simulink model "Simulink"  (R2019b)
settings: Solver=FixedStepAuto  StartTime=0.0  StopTime=5  FixedStep=0.001  RelTol=1e-3
values from neighbouring files (symbols this model uses):
  Awn0 = [0 1; -(wn0^2) -2*wn0*ounce]    [Autonomous_system_simulation.m]    (also in Autonomous_system_simulation_wsimulink.m)
  Awn1 = [0 1; -(wn1^2) -2*wn1*ounce]    [Autonomous_system_simulation.m]    (also in Autonomous_system_simulation_wsimulink.m)
  Awn2 = [0 1; -(wn2^2) -2*wn2*ounce]    [Autonomous_system_simulation.m]    (also in Autonomous_system_simulation_wsimulink.m)
  Awn3 = [0 1; -(wn3^2) -2*wn3*ounce]    [Autonomous_system_simulation.m]    (also in Autonomous_system_simulation_wsimulink.m)
  Cwn0 = [1 0; 0 1]    [Autonomous_system_simulation.m]    (also in Autonomous_system_simulation_wsimulink.m)
  Cwn2 = [1 0; 0 1]    [Autonomous_system_simulation.m]    (also in Autonomous_system_simulation_wsimulink.m)
  Cwn3 = [1 0; 0 1]    [Autonomous_system_simulation.m]    (also in Autonomous_system_simulation_wsimulink.m)
  Dwn0 = [0; 0]    [Autonomous_system_simulation.m]    (also in Autonomous_system_simulation_wsimulink.m)
  Gwn0 = [0; wn0^2]    [Autonomous_system_simulation.m]    (also in Autonomous_system_simulation_wsimulink.m)
  R = eye(2, 2)    [Autonomous_system_simulation.m]    (also in Autonomous_system_simulation_wsimulink.m)
undefined symbols (not defined in the file or in its folder): Continuous, Time
libraries: ctrlSharedLib x3
settings Model: Creator=HP  LastModifiedBy=Bekircan Keceoglu
settings DataIOCC: ReturnWorkspaceOutputs=off
settings DebuggingCC: ArithmeticOperatorsInVariantConditions=warning
settings SFSimCC: CustomCodeUndefinedFunction=UseInterfaceOnly

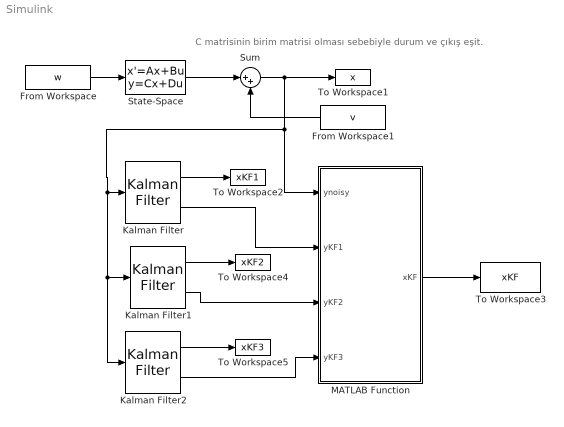
== system Simulink ==
  note: C matrisinin birim matrisi olması sebebiyle durum ve çıkış eşit.
  From Workspace : FromWorkspace  VariableName=w
  From Workspace1 : FromWorkspace  VariableName=v
  Kalman Filter : ctrlSharedLib/Kalman Filter  TimeDomain=Continuous-Time  UseCurrentEstimator=on  ModelSource=Individual A, B, C, D matrices  ModelSourceVariable=ss(0.95,1,1,0,1)  A=Awn1  B=[0;0.25]  C=Awn1  D=[0;0]  NumberOfStates=1  NumberOfInputs=1  NumberOfOutputs=1  InitialEstimateSource=Dialog  X0=0  P0=10  UseK=off  UseGH=on  NumberOfProcessNoiseInputs=1  G=Gwn1  TimeInvariantG=on  H=0  TimeInvariantH=on  Q=Q  TimeInvariantQ=on  R=R  TimeInvariantR=on  N=0  TimeInvariantN=on  AddInputPort=off  AddEnablePort=off  OutputEstimatedY=on  OutputP=off  Ts=-1
      settings: SourceProductBaseCode=CT
  Kalman Filter1 : ctrlSharedLib/Kalman Filter  TimeDomain=Continuous-Time  UseCurrentEstimator=on  ModelSource=Individual A, B, C, D matrices  ModelSourceVariable=ss(0.95,1,1,0,1)  A=Awn2  B=[0;100]  C=Cwn2  D=[0;0]  NumberOfStates=1  NumberOfInputs=1  NumberOfOutputs=1  InitialEstimateSource=Dialog  X0=0  P0=10  UseK=off  UseGH=on  NumberOfProcessNoiseInputs=1  G=Gwn2  TimeInvariantG=on  H=0  TimeInvariantH=on  Q=Q  TimeInvariantQ=on  R=R  TimeInvariantR=on  N=0  TimeInvariantN=on  AddInputPort=off  AddEnablePort=off  OutputEstimatedY=on  OutputP=off  Ts=-1
      settings: SourceProductBaseCode=CT
  Kalman Filter2 : ctrlSharedLib/Kalman Filter  TimeDomain=Continuous-Time  UseCurrentEstimator=on  ModelSource=Individual A, B, C, D matrices  ModelSourceVariable=ss(0.95,1,1,0,1)  A=Awn3  B=[0;625]  C=Cwn3  D=[0;0]  NumberOfStates=1  NumberOfInputs=1  NumberOfOutputs=1  InitialEstimateSource=Dialog  X0=0  P0=10  UseK=off  UseGH=on  NumberOfProcessNoiseInputs=1  G=Gwn3  TimeInvariantG=on  H=0  TimeInvariantH=on  Q=Q  TimeInvariantQ=on  R=R  TimeInvariantR=on  N=0  TimeInvariantN=on  AddInputPort=off  AddEnablePort=off  OutputEstimatedY=on  OutputP=off  Ts=-1
      settings: SourceProductBaseCode=CT
  MATLAB Function : MATLAB Function  TreatAsAtomicUnit=on
  State-Space : StateSpace  A=Awn0  B=Gwn0  C=Cwn0  D=Dwn0  InitialCondition=[1;10]
  Sum : Sum  Inputs=|++
  To Workspace1 : ToWorkspace  VariableName=x  SaveFormat=Timeseries  SampleTime=-1
  To Workspace2 : ToWorkspace  VariableName=xKF1  SaveFormat=Timeseries  SampleTime=-1
  To Workspace3 : ToWorkspace  VariableName=xKF  SaveFormat=Timeseries  SampleTime=-1
  To Workspace4 : ToWorkspace  VariableName=xKF2  SaveFormat=Timeseries  SampleTime=-1
  To Workspace5 : ToWorkspace  VariableName=xKF3  SaveFormat=Timeseries  SampleTime=-1
  wires:
  From Workspace/1 -> State-Space/1
  State-Space/1 -> Sum/1
  From Workspace1/1 -> Sum/2
  MATLAB Function/1(xKF) -> To Workspace3/1
  Sum/1 -> To Workspace1/1, MATLAB Function/1(ynoisy), Kalman Filter2/1, Kalman Filter1/1, Kalman Filter/1
  Kalman Filter/1 -> To Workspace2/1
  Kalman Filter1/1 -> To Workspace4/1
  Kalman Filter2/1 -> To Workspace5/1
  Kalman Filter/2 -> MATLAB Function/2(yKF1)
  Kalman Filter1/2 -> MATLAB Function/3(yKF2)
  Kalman Filter2/2 -> MATLAB Function/4(yKF3)

== matlab function Simulink/MATLAB Function ==
  data: ynoisy input; xKF output; yKF1 input; yKF2 input; yKF3 input
function xKF= decision_maker(ynoisy, yKF1, yKF2, yKF3)

% init xKF
xKF = [0; 0];

% error = (filterO(1) - systemO(1))^2 + (filterO(2) - systemO(2))^2 
eKF1 = (yKF1(1) - ynoisy(1))^2 + (yKF1(2) - ynoisy(2))^2 ;
eKF2 = (yKF2(1) - ynoisy(1))^2 + (yKF2(2) - ynoisy(2))^2 ;
eKF3 = (yKF3(1) - ynoisy(1))^2 + (yKF3(2) - ynoisy(2))^2 ;

% find min error
if ( eKF1 < eKF2 && eKF1 < eKF3 )
    xKF(1) = yKF1(1);
    xKF(2) = yKF1(2);
elseif ( eKF2 < eKF1 && eKF2 < eKF3 )
    xKF(1) = yKF2(1);
    xKF(2) = yKF2(2);
elseif ( eKF3 < eKF1 && eKF3 < eKF2 )
    xKF(1) = yKF3(1);
    xKF(2) = yKF3(2);
end
    
end
